simulink library "lib_controls"  (Simulink 7.9)
settings: Solver=ode45  SolverMode=SingleTasking  StartTime=0.0  StopTime=10.0  RelTol=1e-3
undefined symbols (not defined in the file or in its folder): amb_tmp, cs_charge_deplete_bool, cs_charge_pwr, cs_charge_trq, cs_clt_tmp, cs_decel_fc_off, cs_decel_regen_threshold, cs_dl_assist_trq_threshold, cs_dl_regen_trq_threshold, cs_electric_decel_spd, cs_electric_launch_spd, cs_electric_launch_spd_hi, cs_electric_launch_spd_lo, cs_eng_min_spd, cs_eng_on_soc, cs_fc_init_state, cs_fc_max_pwr_frac, cs_fc_min_pwr_frac, cs_fc_on, cs_fc_pwr_opt, cs_fc_spd_opt, cs_fuzzy_fuel_mode, cs_hi_soc, cs_hi_trq_frac, cs_lo_soc, cs_lo_trq_frac, cs_max_gc_spd, cs_max_pwr, cs_max_pwr_fall_rate, cs_max_pwr_rise_rate, cs_mc_assist_max_frac, cs_mc_assist_min_frac, cs_mc_assist_slope, cs_mc_regen_max_frac, cs_mc_regen_min_frac, cs_mc_regen_slope, cs_mean_eff, cs_mean_eff_bool, cs_min_gc_spd, cs_min_off_time, cs_min_pwr, cs_min_trq_frac, cs_mph_avg_time, cs_off_trq_frac, cs_plot_output, cs_pwr, cs_regen_avg_time, cs_scale_factor, cs_shutoff, cs_soc_range, cs_spd, cs_target_soc, cs_trq_to_soc_factor, cvt_locus_pwr, cvt_locus_spd, cyc_mph, enable_sim_stop_distance, enable_sim_stop_max_spd, enable_sim_stop_speed, enable_sim_stop_time ... (+110)
libraries: lib_controls x124, simulink3 x13, simulink x5, lib_etc x1
(part 8 of 17)

== system lib_controls/<vc> series/gearbox control for series  HV and EV ==
  note: default gear number
      | calculation
  note: default shifting
      | calculation
  note: default gear ratio
      | calculation
  note: local GOTO blocks:
  gb_trq_out_r : Inport
  gb_spd_out_r : Inport  Port=2
  prev. Pout/Pin : Inport  Port=3
  tires are at traction limit : Inport  Port=4
  Block NOTES : Subsystem
      mask Display: disp('Block\nNOTES')
  Constant : Constant
  Constant14 : Constant  Value=tx_speed_dep
  Constant15 : Constant  Value=tx_speed_dep
  Demux : Demux  Outputs=2
  Fcn : Fcn  Expr=1/u
  Fcn1 : Fcn  Expr=1/u
  Gain1 : Gain  Gain=-1  SaturateOnIntegerOverflow=on  OutDataTypeStr=Inherit: Same as input  ParamDataTypeStr=Inherit: Same as input
  MOTOR torque capability : Lookup  InputValues=mc_map_spd*mc_spd_scale  Table=mc_max_trq*mc_trq_scale+eps  SaturateOnIntegerOverflow=on
  Mux : Mux  Inputs=2
  Product2 : Product  Inputs=*/  SaturateOnIntegerOverflow=on  RndMeth=Zero  InputSameDT=on  OutDataTypeStr=Inherit: Same as first input
  Product3 : Product  SaturateOnIntegerOverflow=on  RndMeth=Zero  InputSameDT=on  OutDataTypeStr=Inherit: Same as first input
  Rate Limiter : RateLimiter  RisingSlewLimit=1/(gb_shift_delay+eps)  FallingSlewLimit=-1/(gb_shift_delay+eps)
  Saturation : Saturate  UpperLimit=1  LowerLimit=0.2
  Saturation1 : Saturate  UpperLimit=gb_gears_num  LowerLimit=1
  Speed Dependent Shifting : lib_controls/SubSystem/Speed Dependent Shifting
      settings: RTWFcnNameOpts=Auto  RTWFileNameOpts=Auto
  Switch : Switch  Threshold=eps  SaturateOnIntegerOverflow=on  InputSameDT=on
  Switch3 : Switch  Threshold=0.5  SaturateOnIntegerOverflow=on  InputSameDT=on
  Switch4 : Switch  Threshold=0.5  SaturateOnIntegerOverflow=on  InputSameDT=on
  allow downshift? : Subsystem
  current gear number : Sum  SaturateOnIntegerOverflow=on  InputSameDT=on  OutDataTypeStr=Inherit: Same as first input
  delta gear number : Switch  Threshold=eps  SaturateOnIntegerOverflow=on  InputSameDT=on
  downshift  command : Subsystem
  gb_spd_in_r : Product  SaturateOnIntegerOverflow=on  RndMeth=Zero  InputSameDT=on  OutDataTypeStr=Inherit: Same as first input
  gear ratio : Lookup  InputValues=[1:length(gb_ratio)]  Table=gb_ratio  SaturateOnIntegerOverflow=on
  gear ratio1 : Lookup  InputValues=[1:length(gb_ratio)]  Table=gb_ratio  SaturateOnIntegerOverflow=on
  gearbox speed estimator : Subsystem
  load=T/ (maxT at spd) : Saturate  UpperLimit=1  LowerLimit=0
  prev gear number : Memory  X0=1
  prev gear ratio : Memory  X0=gb_ratio(1)
  shifting1 : Subsystem
  upshift  command : Subsystem
  ~gb_trq_in_r : Product  Inputs=3  SaturateOnIntegerOverflow=on  RndMeth=Zero  InputSameDT=on  OutDataTypeStr=Inherit: Same as first input
  "gear number, out" : Outport  InitialOutput=0
  "gear ratio, out" : Outport  Port=2  InitialOutput=0
  "shifting, out" : Outport  Port=3  InitialOutput=0
  wires:
  gearbox speed estimator/1(Out1) -> MOTOR torque capability/1, downshift  command/3(engine speed), upshift  command/3(engine speed)
  gb_spd_in_r/1 -> gearbox speed estimator/1(gb_spd_in_r if no gear change)
  current gear number/1 -> Saturation1/1
  Saturation/1 -> Fcn/1
  prev. Pout/Pin/1 -> Saturation/1
  gb_trq_out_r/1 -> ~gb_trq_in_r/1
  upshift  command/1(command) -> delta gear number/1, delta gear number/2
  gear ratio/1 -> prev gear ratio/1
  Rate Limiter/1 -> gear ratio/1
  gb_spd_out_r/1 -> gb_spd_in_r/1
  downshift  command/1(command) -> Gain1/1
  Gain1/1 -> Product3/2
  Product3/1 -> delta gear number/3
  allow downshift?/1(allow shift) -> Product3/1
  prev gear ratio/1 -> Fcn1/1, gb_spd_in_r/2
  delta gear number/1 -> current gear number/2
  Fcn1/1 -> ~gb_trq_in_r/3
  MOTOR torque capability/1 -> Product2/2
  Product2/1 -> load=T/ (maxT at spd)/1
  ~gb_trq_in_r/1 -> Product2/1
  Fcn/1 -> ~gb_trq_in_r/2
  load=T/ (maxT at spd)/1 -> Switch/3
  tires are at traction limit/1 -> Switch/2
  Constant/1 -> Switch/1
  Switch/1 -> upshift  command/2(engine load), downshift  command/2(engine load)
  Saturation1/1 -> prev gear number/1, gear ratio1/1, shifting1/1(gear number), Rate Limiter/1, [def_gear_num]
  prev gear number/1 -> allow downshift?/1(prev gearnum), upshift  command/1(prev gear number), downshift  command/1(prev gear number), current gear number/1
  Constant14/1 -> Switch3/2
  [def_gear_num] -> Switch3/3
  Constant15/1 -> Switch4/2
  [spd_dep_muxed] -> Switch4/1
  Mux/1 -> Switch4/3
  [def_gear_ratio] -> Mux/1
  [def_shifting] -> Mux/2
  Switch4/1 -> Demux/1
  [spd_dep_gear_num] -> Switch3/1
  [v_req_limited] -> Speed Dependent Shifting/1
  Speed Dependent Shifting/1 -> [spd_dep_muxed]
  Speed Dependent Shifting/2 -> [spd_dep_gear_num]
  Demux/1 -> "gear ratio, out"/1
  Demux/2 -> "shifting, out"/1
  Switch3/1 -> "gear number, out"/1
  gear ratio1/1 -> [def_gear_ratio]
  shifting1/1(out_1) -> [def_shifting]

== system lib_controls/<vc> series/key_on ==
  Clock : Clock
  Fcn1 : Fcn  Expr=rem(u[1],period)
  Look-Up Table : Lookup  InputValues=t  Table=y  SaturateOnIntegerOverflow=on
  out_1 : Outport  InitialOutput=0
  wires:
  Look-Up Table/1 -> out_1/1
  Clock/1 -> Fcn1/1
  Fcn1/1 -> Look-Up Table/1

== system lib_controls/<vc> series/motor controller logic ==
  bus voltage : Inport
  req'd input power (W) : Inport  Port=2
  req'd output spd (rad/s) : Inport  Port=3
  shifting : Inport  Port=4
  Abs : Abs  SaturateOnIntegerOverflow=on
  Abs1 : Abs  SaturateOnIntegerOverflow=on
  Block NOTES : Subsystem
      mask Display: disp('Block\nNOTES')
  Constant : Constant  Value=mc_max_crrnt
  Constant1 : Constant  Value=0.001
  Constant2 : Constant  Value=0
  Logical Operator1 : Logic  Operator=NOT  Inputs=1
  Memory : Memory  X0=ess_module_num*mean(ess_voc(1,:))
  MinMax : MinMax  Inputs=2  SaturateOnIntegerOverflow=on  InputSameDT=on
  Product1 : Product  SaturateOnIntegerOverflow=on  RndMeth=Zero  InputSameDT=on  OutDataTypeStr=Inherit: Same as first input
  Relational Operator : RelationalOperator  Operator=<=  InputSameDT=on
  Relational Operator2 : RelationalOperator  Operator===  InputSameDT=on
  Sign : Subsystem
      mask Type: Sign
      mask Description: y = sign(x)
      mask Help: Sign Function:\n\t\t\ty = 1 if x > 0\n\t\t\ty = 0 if x = 0\n\t\t\ty = -1 if x < 0
      mask Display: plot(-50,-50,50,50,[-50,50],[0,0],[0,0],[-50,50],[-40,0],[-30,-30],[0,40],[30,30])
  Switch : Switch  Threshold=eps  SaturateOnIntegerOverflow=on  InputSameDT=on
  current-limited power : Product  SaturateOnIntegerOverflow=on  RndMeth=Zero  InputSameDT=on  OutDataTypeStr=Inherit: Same as first input
  true if motor should be shut down : Logic  Operator=OR
  req'd input power (W)1 : Outport  InitialOutput=0
  tag scope: mc_crrnt_limited=global
  wires:
  Abs1/1 -> Relational Operator/1
  true if motor should be shut down/1 -> Logical Operator1/1
  shifting/1 -> true if motor should be shut down/2
  Logical Operator1/1 -> Switch/2
  Constant/1 -> Product1/2
  Abs/1 -> MinMax/2
  Sign/1(out_1) -> current-limited power/2
  Constant2/1 -> Switch/3
  Switch/1 -> req'd input power (W)1/1
  current-limited power/1 -> Switch/1
  Product1/1 -> Relational Operator2/1, MinMax/1
  MinMax/1 -> current-limited power/1, Relational Operator2/2
  Relational Operator2/1 -> [mc_crrnt_limited]
  Relational Operator/1 -> true if motor should be shut down/1
  Constant1/1 -> Relational Operator/2
  req'd output spd (rad/s)/1 -> Abs1/1
  bus voltage/1 -> Memory/1
  Memory/1 -> Product1/1
  req'd input power (W)/1 -> Abs/1, Sign/1(in_1)

== system lib_controls/<vc> series/series 'clutch' control ==
  engine on : Inport
  Block NOTES : Subsystem
      mask Display: disp('Block\nNOTES')
  Clock : Clock
  Constant6 : Constant
  Constant7 : Constant  Value=3
  Memory1 : Memory  X0=cyc_mph(1,2)>0
  Memory2 : Memory  X0=-1
  Sum : Sum  Inputs=+-  SaturateOnIntegerOverflow=on  InputSameDT=on  OutDataTypeStr=Inherit: Same as first input
  Switch : Switch  Threshold=eps  SaturateOnIntegerOverflow=on  InputSameDT=on
  Switch1 : Switch  Threshold=0.5  SaturateOnIntegerOverflow=on  InputSameDT=on
  Transport Delay : TransportDelay  DelayTime=0.5
  clutch slipping1 : Logic
  clutch slipping2 : Logic
  clutch state : Outport
  wires:
  engine on/1 -> clutch slipping2/1, Transport Delay/1, Memory1/1, clutch slipping1/1
  Sum/1 -> Switch1/2
  Memory2/1 -> Sum/2
  Clock/1 -> Memory2/1, Sum/1
  clutch slipping2/1 -> Switch1/3
  Transport Delay/1 -> clutch slipping2/2
  clutch slipping1/1 -> Switch1/1
  Constant6/1 -> Switch/3
  Switch/1 -> clutch state/1
  Switch1/1 -> Switch/2
  Constant7/1 -> Switch/1
  Memory1/1 -> clutch slipping1/2

== system lib_controls/Adaptive control strategy <cs>/Delta SOC expected from regen ==
  "trq and spd req'd into clutch (N*m, rad/s)" : Inport
  "  1" : Constant  Value=0
  " 2" : Constant  Value=0
  Delta SOC : Sum  Inputs=-+  SaturateOnIntegerOverflow=on  InputSameDT=on  OutDataTypeStr=Inherit: Same as first input
  Logical Operator : Logic
  Memory1 : Memory  X0=ess_init_soc
  "Regen  (Tmc<0,  but Tfc<=0)" : Switch  Threshold=eps  SaturateOnIntegerOverflow=on  InputSameDT=on
  Regen flag conditions : Constant  Value=0
  Relational Operator : RelationalOperator  Operator=<=  InputSameDT=on
  Relational Operator1 : RelationalOperator  Operator=<  InputSameDT=on
  Saturation : Saturate  UpperLimit=1  LowerLimit=0
  Subsystem : Subsystem  mask(Running Average){n=cs_regen_avg_time}
      mask prompts: n "Averaging Time (s)"
      mask help: Running Average
      mask Help: Output is the average of the last (Averaging Time) seconds of input.
      mask Display: disp('Running\nAverage')
  trq : Selector  InputPortWidth=2  IndexOptions=Index vector (dialog)  Indices=1  OutputSizes=1
  Delta SOC regen : Outport
  wires:
  Delta SOC/1 -> Saturation/1
  "Regen  (Tmc<0,  but Tfc<=0)"/1 -> Subsystem/1(in_1)
  Subsystem/1(out_1) -> Delta SOC regen/1
  Logical Operator/1 -> "Regen  (Tmc<0,  but Tfc<=0)"/2
  [SOC] -> Delta SOC/2, Memory1/1
  Memory1/1 -> Delta SOC/1
  Saturation/1 -> "Regen  (Tmc<0,  but Tfc<=0)"/1
  "trq and spd req'd into clutch (N*m, rad/s)"/1 -> trq/1
  "  1"/1 -> "Regen  (Tmc<0,  but Tfc<=0)"/3
  trq/1 -> Relational Operator/1
  Relational Operator/1 -> Logical Operator/2
  Relational Operator1/1 -> Logical Operator/1
  Regen flag conditions/1 -> Relational Operator/2
  " 2"/1 -> Relational Operator1/2
  [mc_trq_out_a] -> Relational Operator1/1

== system lib_controls/Adaptive control strategy <cs>/Finds operation  point - energy/emissions  weighting ==
  "trq and spd req'd into clutch (N*m, rad/s)" : Inport
  Delta SOC expected from regen : Inport  Port=2
  Memory : Memory  X0=amb_tmp
  Memory1 : Memory  X0=amb_tmp
  Memory2 : Memory  X0=amb_tmp
  Minimize the  energy used  and emissions : Subsystem
  Mux2 : Mux  Inputs=7
  Subsystem : Subsystem  mask(Running Average){n=cs_mph_avg_time}
      mask prompts: n "Averaging Time (s)"
      mask help: Running Average
      mask Help: Output is the average of the last (Averaging Time) seconds of input.
      mask Display: disp('Running\nAverage')
  total fuel used (gal)1 : ToWorkspace  VariableName=cs_DeltaSOC_regen
      settings: MaxDataPoints=50000
  trq req'd from  engine (N*m) : Outport
  wires:
  Delta SOC expected from regen/1 -> total fuel used (gal)1/1, Mux2/2
  [ex_cat_tmp] -> Memory/1
  Memory/1 -> Mux2/6
  [cyc_mph_r] -> Subsystem/1(in_1)
  Subsystem/1(out_1) -> Mux2/4
  [SOC] -> Mux2/3
  [ess_tmp] -> Memory2/1
  Memory2/1 -> Mux2/7
  Mux2/1 -> Minimize the  energy used  and emissions/1(input vector)
  Minimize the  energy used  and emissions/1(Tfc) -> trq req'd from  engine (N*m)/1
  [fc_clt_tmp] -> Memory1/1
  Memory1/1 -> Mux2/5
  "trq and spd req'd into clutch (N*m, rad/s)"/1 -> Mux2/1

== system lib_controls/Fuzzy Logic control strategy <cs>/Block NOTES ==
  note: Where TLOAD is the load required from the drive cycle due to acceleration, drag, road grade, etc., and
      | TICE_Set is the desired output torque of the ICE.  The controller outputs the change of the throttle command.
  note: Due to the highly nonlinear, time varying nature of the plant, the control strategy will be
      |  implemented with the use of a fuzzy logic controller (FLC). The FLC will use two
      | inputs:  the battery pack SOC and the desired ICE torque. Based on the above inputs,
      | the ICE operating point is set (according to the MODE selected). Along the simulation,
      | in the reverse loop, the desired e-machine torque is calculated from the
      | following equation.
      |
      | TEM_Desired = TLOAD - TICE_Set
  note: The idea behind the Fuzzy Logic control strategy is to let the ICE run at an operating point
      | that consumes less than x gram of fuel per second at all operating conditions (FUSE USE MODE) or to
      | operate about a preak efficiency point (EFFICIENCY MODE).  Since an Electric Machine is available
      | to load-level, the HEV can use its e-machine to force the engine to operate in a region that consumes less fuel,
      | while maintaining  the state of charge (SOC) of the battery pack over the  majority of the drive cycle.
      | This is achieved by  using to E-Machine to compensate for the dearth in Torque required to meet the road load.
  note: This Block contains the Fuzzy Logic Control Strategy to control a parallel hybrid configuration.
      |
      | A standard set of inputs (SoC and ICE torque required) are input in the beginning. Then scaling is done
      | to the inputs to reflect the input membership functions. Likewise, the outputs are scaled based on the no. of output
      | membership functions. The above block diagram also calls the M-Function which contains the rules.

== system lib_controls/Fuzzy Logic control strategy <cs>/Fuzzy logic Code ==
  note: FUZZY LOGIC CODE
  Torque : Inport
  SoC : Inport  Port=2
  Block NOTES : Subsystem
      mask Display: disp('Block\nNOTES')
  Fuel use  or Efficieny : Switch  Threshold=eps  SaturateOnIntegerOverflow=on  InputSameDT=on
  MATLAB Fcn EFFICIENCY MODE : MATLABFcn  MATLABFcn=mfuzzy_eff_mode(u(1),u(2))  OutputDimensions=1
  MATLAB Fcn FUEL USE MODE : MATLABFcn  MATLABFcn=mfuzzy_fuel_mode(u(1),u(2))  OutputDimensions=1
  Mode switcher : Constant  Value=cs_fuzzy_fuel_mode
  Mux : Mux  Inputs=2
  delta  alpha : Outport
  wires:
  Mux/1 -> MATLAB Fcn FUEL USE MODE/1, MATLAB Fcn EFFICIENCY MODE/1
  Torque/1 -> Mux/1
  SoC/1 -> Mux/2
  Mode switcher/1 -> Fuel use  or Efficieny/2
  Fuel use  or Efficieny/1 -> delta  alpha/1
  MATLAB Fcn FUEL USE MODE/1 -> Fuel use  or Efficieny/1
  MATLAB Fcn EFFICIENCY MODE/1 -> Fuel use  or Efficieny/3

== system lib_controls/Fuzzy Logic control strategy <cs>/Input Scaling ==
  note: INPUT SCALING
  note: STANDARD INPUTS
  Torque required : Inport
  " 2" : Sum  SaturateOnIntegerOverflow=on  InputSameDT=on  OutDataTypeStr=Inherit: Same as first input
  " 3" : Sum  Inputs=+-  SaturateOnIntegerOverflow=on  InputSameDT=on  OutDataTypeStr=Inherit: Same as first input
  " 5" : Sum  SaturateOnIntegerOverflow=on  InputSameDT=on  OutDataTypeStr=Inherit: Same as first input
  " 6" : Sum  SaturateOnIntegerOverflow=on  InputSameDT=on  OutDataTypeStr=Inherit: Same as first input
  " 7" : Sum  Inputs=++-  SaturateOnIntegerOverflow=on  InputSameDT=on  OutDataTypeStr=Inherit: Same as first input
  Block NOTES : Subsystem
      mask Display: disp('Block\nNOTES')
  Constant5 : Constant  Value=5
  Constant6 : Constant
  Constant7 : Constant  Value=5
  Constant8 : Constant  Value=6
  Constant9 : Constant  Value=10e4*eps
  Product8 : Product  Inputs=**/  SaturateOnIntegerOverflow=on  RndMeth=Zero  InputSameDT=on  OutDataTypeStr=Inherit: Same as first input
  Relational Operator : RelationalOperator  Operator=<=  InputSameDT=on
  Saturation 1-11 : Saturate  UpperLimit=11  LowerLimit=1
  "Saturation 1-11 " : Saturate  UpperLimit=11  LowerLimit=1
  SoC scaling function 1-11 : Fcn  Expr=10*(u-cs_hi_soc)/(cs_hi_soc-cs_lo_soc)+11
  Switch1 : Switch  Threshold=eps  SaturateOnIntegerOverflow=on  InputSameDT=on
  Target ICE Line : Lookup  InputValues=fc_map_spd*fc_spd_scale  Table=flc_target*fc_trq_scale  SaturateOnIntegerOverflow=on
  epsilon : Constant  Value=eps
  max_torque lookup : Lookup  InputValues=fc_map_spd*fc_spd_scale  Table=fc_max_trq*fc_trq_scale  SaturateOnIntegerOverflow=on
  trouble : Product  Inputs=**/  SaturateOnIntegerOverflow=on  RndMeth=Zero  InputSameDT=on  OutDataTypeStr=Inherit: Same as first input
  Torque : Outport
  SoC : Outport  Port=2
  tag scope: FLC1=global
  wires:
  Relational Operator/1 -> Switch1/2
  Product8/1 -> " 2"/1
  Constant6/1 -> " 2"/2
  " 2"/1 -> Switch1/1
  " 3"/1 -> trouble/1
  Constant7/1 -> trouble/2
  Constant8/1 -> " 5"/2
  trouble/1 -> " 5"/1
  [SOC] -> SoC scaling function 1-11/1
  Saturation 1-11/1 -> SoC/1
  " 5"/1 -> Switch1/3
  "Saturation 1-11 "/1 -> Torque/1
  Constant5/1 -> Product8/2
  Constant9/1 -> " 7"/2
  epsilon/1 -> " 6"/1
  " 6"/1 -> Product8/3
  " 7"/1 -> trouble/3
  [engine_rpm] -> Target ICE Line/1, max_torque lookup/1
  SoC scaling function 1-11/1 -> Saturation 1-11/1
  Switch1/1 -> "Saturation 1-11 "/1
  max_torque lookup/1 -> " 7"/1
  Torque required/1 -> Product8/1, Relational Operator/1, " 3"/1
  Target ICE Line/1 -> [FLC1], Relational Operator/2, " 6"/2, " 3"/2, " 7"/3

== system lib_controls/Fuzzy Logic control strategy <cs>/Output scaling ==
  note: OUTPUT SCALING
  "delta alpha " : Inport
  " " : Sum  Inputs=+-  SaturateOnIntegerOverflow=on  InputSameDT=on  OutDataTypeStr=Inherit: Same as first input
  " 1" : Sum  Inputs=+-  SaturateOnIntegerOverflow=on  InputSameDT=on  OutDataTypeStr=Inherit: Same as first input
  " 2" : Sum  SaturateOnIntegerOverflow=on  InputSameDT=on  OutDataTypeStr=Inherit: Same as first input
  " 3" : Sum  Inputs=+-  SaturateOnIntegerOverflow=on  InputSameDT=on  OutDataTypeStr=Inherit: Same as first input
  Block NOTES : Subsystem
      mask Display: disp('Block\nNOTES')
  Constant : Constant  Value=6
  Constant1 : Constant
  Constant2 : Constant  Value=5
  Constant3 : Constant  Value=6
  Constant4 : Constant  Value=5
  Product4 : Product  SaturateOnIntegerOverflow=on  RndMeth=Zero  InputSameDT=on  OutDataTypeStr=Inherit: Same as first input
  Product5 : Product  Inputs=*/  SaturateOnIntegerOverflow=on  RndMeth=Zero  InputSameDT=on  OutDataTypeStr=Inherit: Same as first input
  Product6 : Product  SaturateOnIntegerOverflow=on  RndMeth=Zero  InputSameDT=on  OutDataTypeStr=Inherit: Same as first input
  Product7 : Product  Inputs=*/  SaturateOnIntegerOverflow=on  RndMeth=Zero  InputSameDT=on  OutDataTypeStr=Inherit: Same as first input
  Relational Operator : RelationalOperator  Operator=<=  InputSameDT=on
  Saturation 1-11 : Saturate  UpperLimit=11  LowerLimit=1
  Saturation4 : Saturate  UpperLimit=max(fc_max_trq*fc_trq_scale)  LowerLimit=0
  Switch1 : Switch  Threshold=eps  SaturateOnIntegerOverflow=on  InputSameDT=on
  max_torque lookup : Lookup  InputValues=fc_map_spd*fc_spd_scale  Table=fc_max_trq*fc_trq_scale  SaturateOnIntegerOverflow=on
  ICE Torque command : Outport
  wires:
  Constant/1 -> Relational Operator/2
  Constant1/1 -> " "/2
  Saturation 1-11/1 -> Relational Operator/1, " "/1
  " "/1 -> Product4/2
  Product4/1 -> Product5/1
  Constant2/1 -> Product5/2
  [FLC1] -> Product4/1, " 2"/2, " 3"/2
  "delta alpha "/1 -> " 1"/1, Saturation 1-11/1
  Constant3/1 -> " 1"/2
  " 1"/1 -> Product6/1
  " 3"/1 -> Product6/2
  Product6/1 -> Product7/1
  Constant4/1 -> Product7/2
  Product5/1 -> Switch1/1
  Relational Operator/1 -> Switch1/2
  " 2"/1 -> Switch1/3
  Product7/1 -> " 2"/1
  Switch1/1 -> Saturation4/1
  Saturation4/1 -> ICE Torque command/1
  [engine_rpm] -> max_torque lookup/1
  max_torque lookup/1 -> " 3"/1

== system lib_controls/Fuzzy Logic control strategy <cs>/help ==

== system lib_controls/Fuzzy Logic control strategy with Emissions <cs>/Block NOTES ==
  note: The Fuzzy Control Block takes in the torque and speed requested by the clutch (sink) and calculates
      | the torque split between the ICE and the Motor. The fuzzy logic algorithm sets a base (optimal)
      | operating point of the ICE and modifies the actual operating point about the optimal, based on
      | the actual torque request and the battery State of Charge (SOC). Finally, a torque request is sent to the
      | ICE and the motor buffers the remaining torque (positive or negative).

== system lib_controls/Fuzzy Logic control strategy with Emissions <cs>/Fuzzy logic Code ==
  note: FUZZY LOGIC CODE
  Torque : Inport
  SoC : Inport  Port=2
  Block NOTES : Subsystem
      mask Display: disp('Block\nNOTES')
  "MATLAB Fcn GPS " : MATLABFcn  MATLABFcn=mfuzzy_emissions(u(1),u(2))  OutputDimensions=1
  Mux : Mux  Inputs=2
  delta  alpha : Outport
  wires:
  Mux/1 -> "MATLAB Fcn GPS "/1
  Torque/1 -> Mux/1
  "MATLAB Fcn GPS "/1 -> delta  alpha/1
  SoC/1 -> Mux/2

== system lib_controls/Fuzzy Logic control strategy with Emissions <cs>/Input Scaling ==
  note: INPUTS
  note: INPUT SCALING
  note: Engine COLD
  note: Motor Max
      | Torque reached
  note: engine speed
  Torque required : Inport
  " 2" : Sum  SaturateOnIntegerOverflow=on  InputSameDT=on  OutDataTypeStr=Inherit: Same as first input
  " 3" : Sum  Inputs=+-  SaturateOnIntegerOverflow=on  InputSameDT=on  OutDataTypeStr=Inherit: Same as first input
  " 5" : Sum  SaturateOnIntegerOverflow=on  InputSameDT=on  OutDataTypeStr=Inherit: Same as first input
  " 6" : Sum  SaturateOnIntegerOverflow=on  InputSameDT=on  OutDataTypeStr=Inherit: Same as first input
  " 7" : Sum  Inputs=++-  SaturateOnIntegerOverflow=on  InputSameDT=on  OutDataTypeStr=Inherit: Same as first input
  Block NOTES : Subsystem
      mask Display: disp('Block\nNOTES')
  Constant5 : Constant  Value=5
  Constant6 : Constant
  Constant7 : Constant  Value=5
  Constant8 : Constant  Value=6
  Constant9 : Constant  Value=10e4*eps
  Gain : Gain  Gain=vc_fc_warm_tmp_frac  SaturateOnIntegerOverflow=on  OutDataTypeStr=Inherit: Same as input  ParamDataTypeStr=Inherit: Same as input
  MATLAB Fcn Target torque : MATLABFcn  MATLABFcn=fuzzy_target_compute_emissions(u(1),u(2),u(3))  OutputDimensions=1
  Memory : Memory
  Mux : Mux  Inputs=3
  Product8 : Product  Inputs=**/  SaturateOnIntegerOverflow=on  RndMeth=Zero  InputSameDT=on  OutDataTypeStr=Inherit: Same as first input
  Relational Operator : RelationalOperator  Operator=<=  InputSameDT=on
  Relational Operator5 : RelationalOperator  Operator=<  InputSameDT=on
  "Saturation 1-11 " : Saturate  UpperLimit=11  LowerLimit=1
  Switch1 : Switch  Threshold=eps  SaturateOnIntegerOverflow=on  InputSameDT=on
  To Workspace4 : ToWorkspace  VariableName=flc_opt_trq  SampleTime=-1
  To Workspace5 : ToWorkspace  VariableName=flc_max_trq  SampleTime=-1
  epsilon : Constant  Value=eps
  max_torque lookup : Lookup  InputValues=fc_map_spd*fc_spd_scale  Table=fc_max_trq*fc_trq_scale  SaturateOnIntegerOverflow=on
  product : Product  Inputs=**/  SaturateOnIntegerOverflow=on  RndMeth=Zero  InputSameDT=on  OutDataTypeStr=Inherit: Same as first input
  thermostat setting : Constant  Value=fc_tstat
  Torque : Outport
  tag scope: FLC1=global
  wires:
  Switch1/1 -> "Saturation 1-11 "/1
  " 7"/1 -> product/3
  " 6"/1 -> Product8/3
  epsilon/1 -> " 6"/1
  Constant9/1 -> " 7"/2
  Constant5/1 -> Product8/2
  "Saturation 1-11 "/1 -> Torque/1
  " 5"/1 -> Switch1/3
  product/1 -> " 5"/1
  Constant8/1 -> " 5"/2
  Constant7/1 -> product/2
  " 3"/1 -> product/1
  " 2"/1 -> Switch1/1
  Constant6/1 -> " 2"/2
  Product8/1 -> " 2"/1
  Relational Operator/1 -> Switch1/2
  MATLAB Fcn Target torque/1 -> To Workspace4/1, " 7"/3, " 3"/2, " 6"/2, Relational Operator/2, [FLC1]
  [engine_rpm] -> max_torque lookup/1, Mux/3
  Mux/1 -> MATLAB Fcn Target torque/1
  max_torque lookup/1 -> " 7"/1, To Workspace5/1
  Torque required/1 -> " 3"/1, Relational Operator/1, Product8/1
  [mc_trq_limited] -> Memory/1
  thermostat setting/1 -> Gain/1
  Gain/1 -> Relational Operator5/2
  [fc_clt_tmp] -> Relational Operator5/1
  Relational Operator5/1 -> Mux/1
  Memory/1 -> Mux/2

== system lib_controls/Fuzzy Logic control strategy with Emissions <cs>/Output scaling ==
  note: OUTPUT SCALING
  "delta alpha " : Inport
  " " : Sum  Inputs=+-  SaturateOnIntegerOverflow=on  InputSameDT=on  OutDataTypeStr=Inherit: Same as first input
  " 1" : Sum  Inputs=+-  SaturateOnIntegerOverflow=on  InputSameDT=on  OutDataTypeStr=Inherit: Same as first input
  " 2" : Sum  SaturateOnIntegerOverflow=on  InputSameDT=on  OutDataTypeStr=Inherit: Same as first input
  " 3" : Sum  Inputs=+-  SaturateOnIntegerOverflow=on  InputSameDT=on  OutDataTypeStr=Inherit: Same as first input
  Block NOTES : Subsystem
      mask Display: disp('Block\nNOTES')
  Constant : Constant  Value=6
  Constant1 : Constant
  Constant2 : Constant  Value=5
  Constant3 : Constant  Value=6
  Constant4 : Constant  Value=5
  Product4 : Product  SaturateOnIntegerOverflow=on  RndMeth=Zero  InputSameDT=on  OutDataTypeStr=Inherit: Same as first input
  Product5 : Product  Inputs=*/  SaturateOnIntegerOverflow=on  RndMeth=Zero  InputSameDT=on  OutDataTypeStr=Inherit: Same as first input
  Product6 : Product  SaturateOnIntegerOverflow=on  RndMeth=Zero  InputSameDT=on  OutDataTypeStr=Inherit: Same as first input
  Product7 : Product  Inputs=*/  SaturateOnIntegerOverflow=on  RndMeth=Zero  InputSameDT=on  OutDataTypeStr=Inherit: Same as first input
  Relational Operator : RelationalOperator  Operator=<=  InputSameDT=on
  Saturation 1-11 : Saturate  UpperLimit=11  LowerLimit=1
  Saturation4 : Saturate  UpperLimit=max(fc_max_trq*fc_trq_scale)  LowerLimit=0
  Switch1 : Switch  Threshold=eps  SaturateOnIntegerOverflow=on  InputSameDT=on
  max_torque lookup : Lookup  InputValues=fc_map_spd*fc_spd_scale  Table=fc_max_trq*fc_trq_scale  SaturateOnIntegerOverflow=on
  ICE Torque command : Outport
  wires:
  max_torque lookup/1 -> " 3"/1
  [engine_rpm] -> max_torque lookup/1
  Saturation4/1 -> ICE Torque command/1
  Switch1/1 -> Saturation4/1
  Product7/1 -> " 2"/1
  " 2"/1 -> Switch1/3
  Relational Operator/1 -> Switch1/2
  Product5/1 -> Switch1/1
  Constant4/1 -> Product7/2
  Product6/1 -> Product7/1
  " 3"/1 -> Product6/2
  " 1"/1 -> Product6/1
  Constant3/1 -> " 1"/2
  "delta alpha "/1 -> Saturation 1-11/1, " 1"/1
  [FLC1] -> " 3"/2, " 2"/2, Product4/1
  Constant2/1 -> Product5/2
  Product4/1 -> Product5/1
  " "/1 -> Product4/2
  Saturation 1-11/1 -> " "/1, Relational Operator/1
  Constant1/1 -> " "/2
  Constant/1 -> Relational Operator/2

== system lib_controls/Fuzzy Logic control strategy with Emissions <cs>/SoC  ==
  note: soc
  note: cs_hi_soc
  note: cs_lo_soc
  note: BASE SOC LIMITS
      | High= 0. 55
      | Low  = 0.45
  Block NOTES : Subsystem
      mask Display: disp('Block\nNOTES')
  Mux : Mux  Inputs=3
  Saturation 1-11 : Saturate  UpperLimit=11  LowerLimit=1
  SoC scaling function 1-11 : Fcn  Expr=10*(u(1)-u(2))/(u(2)-u(3))+11
  default = 0.45 : Constant  Value=cs_lo_soc
  default = 0.55 : Constant  Value=cs_hi_soc
  SoC : Outport
  wires:
  Mux/1 -> SoC scaling function 1-11/1
  [SOC] -> Mux/1
  default = 0.55/1 -> Mux/2
  default = 0.45/1 -> Mux/3
  SoC scaling function 1-11/1 -> Saturation 1-11/1
  Saturation 1-11/1 -> SoC/1

== system lib_controls/Insight electric assist control strategy <cs> DIRECT SPLIT/1st gear ? ==
  note: 1st Gear
  In 1 : Inport
  In 2 : Inport  Port=2
  Constant : Constant  Value=125
  Constant1 : Constant
  Logical Operator : Logic
  Relational Operator1 : RelationalOperator  Operator===  InputSameDT=on
  Relational Operator2 : RelationalOperator  Operator=<  InputSameDT=on
  Switch11 : Switch  Threshold=eps  SaturateOnIntegerOverflow=on  InputSameDT=on
  Out1 : Outport
  wires:
  In 2/1 -> Switch11/1
  In 1/1 -> Switch11/3
  Constant1/1 -> Relational Operator1/2
  [gear_number] -> Relational Operator1/1
  Switch11/1 -> Out1/1
  Constant/1 -> Relational Operator2/2
  [cs_trq_in_r] -> Relational Operator2/1
  Relational Operator2/1 -> Logical Operator/2
  Logical Operator/1 -> Switch11/2
  Relational Operator1/1 -> Logical Operator/1

== system lib_controls/Insight electric assist control strategy <cs> DIRECT SPLIT/Alternator Function ==
  note: current speed (rad/s)
  note: Torque request
  In1 : Inport
  In2 : Inport  Port=2
  Block NOTES : Subsystem
      mask Display: disp('Block\nNOTES')
  Constant1 : Constant  Value=0
  Constant2 : Constant  Value=0
  Constant3 : Constant  Value=0
  Product : Product  Inputs=*/  SaturateOnIntegerOverflow=on  RndMeth=Zero  InputSameDT=on  OutDataTypeStr=Inherit: Same as first input
  Product1 : Product  Inputs=*/  SaturateOnIntegerOverflow=on  RndMeth=Zero  InputSameDT=on  OutDataTypeStr=Inherit: Same as first input
  Relational Operator1 : RelationalOperator  Operator===  InputSameDT=on
  Relational Operator6 : RelationalOperator  Operator=>  InputSameDT=on
  Sum{2..5} (4 alike) : Sum  Inputs=+-  SaturateOnIntegerOverflow=on  InputSameDT=on  OutDataTypeStr=Inherit: Same as first input
  Sum7 : Sum  Inputs=--  SaturateOnIntegerOverflow=on  InputSameDT=on  OutDataTypeStr=Inherit: Same as first input
  Switch1 : Switch  Threshold=eps  SaturateOnIntegerOverflow=on  InputSameDT=on
  Switch8 : Switch  Threshold=eps  SaturateOnIntegerOverflow=on  InputSameDT=on
  motor/controller input power map (W) only base torque : Lookup2D  RowIndex=mc_map_spd*mc_spd_scale  ColumnIndex=mc_map_trq*mc_trq_scale  Table=mc_inpwr_map*mc_spd_scale*mc_trq_scale  SaturateOnIntegerOverflow=on  InputSameDT=on
  motor/controller input power map (W) with REGEN : Lookup2D  RowIndex=mc_map_spd*mc_spd_scale  ColumnIndex=mc_map_trq*mc_trq_scale  Table=mc_inpwr_map*mc_spd_scale*mc_trq_scale  SaturateOnIntegerOverflow=on  InputSameDT=on
  prevent  divide by zero error : Saturate  UpperLimit=max(fc_spd_scale*fc_map_spd)  LowerLimit=vc_idle_spd
  prevent  divide by zero error2 : Saturate  UpperLimit=max(fc_spd_scale*fc_map_spd)  LowerLimit=vc_idle_spd
  saturation : Saturate  UpperLimit=inf  LowerLimit=0
  Motor torque : Outport
  alternator torque : Outport  Port=2
  wires:
  [acc_elec_pwr_est] -> Product/1
  Relational Operator6/1 -> Switch8/2
  Constant3/1 -> Relational Operator6/2
  prevent  divide by zero error2/1 -> Product1/2, motor/controller input power map (W) only base torque/1, motor/controller input power map (W) with REGEN/1
  [acc_elec_pwr_est] -> Sum5/1
  In2/1 -> prevent  divide by zero error2/1
  Sum2/1 -> motor/controller input power map (W) with REGEN/2, Sum3/1
  In1/1 -> motor/controller input power map (W) only base torque/2, Sum2/1, Switch8/1, Relational Operator6/1, Relational Operator1/1
  Sum5/1 -> saturation/1
  saturation/1 -> Product1/1
  motor/controller input power map (W) with REGEN/1 -> Sum4/2
  Sum4/1 -> Sum5/2
  prevent  divide by zero error/1 -> Product/2
  [engine_rpm] -> prevent  divide by zero error/1
  Switch8/1 -> Motor torque/1
  Product/1 -> Sum2/2, Sum7/2
  Sum7/1 -> alternator torque/1
  Sum3/1 -> Switch8/3
  Product1/1 -> Sum3/2, Sum7/1
  Constant1/1 -> Relational Operator1/2
  Relational Operator1/1 -> Switch1/2
  motor/controller input power map (W) only base torque/1 -> Switch1/3
  Constant2/1 -> Switch1/1
  Switch1/1 -> Sum4/1

== system lib_controls/Insight electric assist control strategy <cs> DIRECT SPLIT/Block NOTES ==
  note: HONDA INSIGHT TORQUE SPLIT CONTROL STRATEGY
      |
      | The Honda Insight Control Startegy is modeled in this block. The Input is the Torque and speed
      | required into the clutch. The electric motor torque contibution is then calculated based on the
      | following parameters:
      | 1. Acceleration torque
      | 2. Deceleration torque
      | 3. 1st gear selection
      | 4. Vehicle speed
      | etc...
      |
      | The electric motor is also the alternator in the vehicle. Thus, it produces the power required by the
      | accessory loads. The remaining is then demanded from the IC Engine. The 2 signals are then
      | sent to the respective blocks in the INSIGHT Model.

== system lib_controls/Insight electric assist control strategy <cs> DIRECT SPLIT/Clutch Engaged ? ==
  note: clutch not
      | disengaged
  note: Any torque
      |  requested from
      | Electric Motor
      | only when
      | clutch engaged
  In1 : Inport
  In2 : Inport  Port=2
  Constant2 : Constant
  Constant3 : Constant
  Constant4 : Constant  Value=0
  Logical Operator : Logic  Operator=NOT
  Relational Operator2 : RelationalOperator  Operator===  InputSameDT=on
  Relational Operator3 : RelationalOperator  Operator===  InputSameDT=on
  Switch2 : Switch  Threshold=eps  SaturateOnIntegerOverflow=on  InputSameDT=on
  Switch3 : Switch  Threshold=eps  SaturateOnIntegerOverflow=on  InputSameDT=on
  Out1 : Outport
  wires:
  Relational Operator2/1 -> Logical Operator/1
  [clutch_state] -> Relational Operator2/1
  Constant2/1 -> Relational Operator2/2
  Constant3/1 -> Relational Operator3/2
  Relational Operator3/1 -> Switch3/2
  Constant4/1 -> Switch3/3
  Switch3/1 -> Switch2/3
  In2/1 -> Switch3/1
  [engine_on] -> Relational Operator3/1
  Logical Operator/1 -> Switch2/2
  In1/1 -> Switch2/1
  Switch2/1 -> Out1/1

== system lib_controls/Insight electric assist control strategy <cs> DIRECT SPLIT/Hard Acceleration ==
  note: Transient = 1
  note: moderate
      | accn
  note: Insight max. effort Torque from motor
      | will be the minimum between
      | {6000 W/shaft_speed} Nm AND
      | the maximum output torque of motor (Nm)
  In1 : Inport
  In2 : Inport  Port=2
  Constant : Constant  Value=125
  Constant1 : Constant  Value=6000*mc_trq_scale
  Constant2 : Constant  Value=max(mc_max_trq)*mc_trq_scale
  Constant6 : Constant  Value=cs_dl_assist_trq_threshold
  Constant7 : Constant  Value=.3
  Define the Assist Characteristics : Fcn  Expr=cs_mc_assist_slope*(u-cs_dl_assist_trq_threshold)+ (cs_mc_assist_min_frac*max(mc_max_trq*mc_trq_scale))
  Derivative : Derivative
  Logical Operator : Logic
  MinMax : MinMax  Inputs=2  SaturateOnIntegerOverflow=on  InputSameDT=on
  Product1 : Product  Inputs=*/  SaturateOnIntegerOverflow=on  RndMeth=Zero  InputSameDT=on  OutDataTypeStr=Inherit: Same as first input
  Relational Operator2 : RelationalOperator  Operator=>  InputSameDT=on
  Relational Operator5 : RelationalOperator  InputSameDT=on
  Relational Operator6 : RelationalOperator  InputSameDT=on
  Saturate motor torque at approx 32% max trq : Saturate  UpperLimit=max(mc_max_trq*mc_trq_scale)*cs_mc_assist_max_frac  LowerLimit=min(mc_max_gen_trq*mc_trq_scale)
  Switch10 : Switch  Threshold=eps  SaturateOnIntegerOverflow=on  InputSameDT=on
  Switch2 : Switch  Threshold=eps  SaturateOnIntegerOverflow=on  InputSameDT=on
  "filter from divide by zero  or negative " : lib_etc/filter from divide by zero  or negative 
      settings: RTWFcnNameOpts=Auto  RTWFileNameOpts=Auto
  Out1 : Outport
  wires:
  Constant7/1 -> Relational Operator6/2
  Derivative/1 -> Relational Operator6/1
  Switch10/1 -> Switch2/3
  In2/1 -> Switch10/3
  Logical Operator/1 -> Switch10/2
  Relational Operator5/1 -> Logical Operator/1
  Relational Operator6/1 -> Logical Operator/2
  Define the Assist Characteristics/1 -> Saturate motor torque at approx 32% max trq/1
  Saturate motor torque at approx 32% max trq/1 -> Switch10/1
  Constant6/1 -> Relational Operator5/2
  In1/1 -> Relational Operator5/1, Define the Assist Characteristics/1, Relational Operator2/1
  [v_req_limited] -> Derivative/1
  Constant/1 -> Relational Operator2/2
  Constant1/1 -> Product1/1
  Relational Operator2/1 -> Switch2/2
  Switch2/1 -> Out1/1
  "filter from divide by zero  or negative "/1 -> Product1/2
  [fc_spd_est] -> "filter from divide by zero  or negative "/1
  MinMax/1 -> Switch2/1
  Product1/1 -> MinMax/2
  Constant2/1 -> MinMax/1

== system lib_controls/Insight electric assist control strategy <cs> DIRECT SPLIT/Hard Deceleration ==
  note: heavy decel
  note: light decel
  In1 : Inport
  Constant3 : Constant  Value=cs_dl_regen_trq_threshold
  Constant4 : Constant  Value=cs_dl_regen_trq_threshold
  Constant5 : Constant  Value=0
  Constant7 : Constant  Value=0
  Define regenerative  capabilities : Fcn  Expr=(u-cs_dl_regen_trq_threshold)*cs_mc_regen_slope + (cs_mc_regen_min_frac*min(mc_max_gen_trq*mc_trq_scale))
  Logical Operator : Logic
  Relational Operator3 : RelationalOperator  Operator=<=  InputSameDT=on
  Relational Operator4 : RelationalOperator  Operator=<  InputSameDT=on
  Relational Operator5 : RelationalOperator  Operator=>  InputSameDT=on
  Saturate motor torque at 100% max regen trq : Saturate  UpperLimit=max(mc_max_trq*mc_trq_scale)  LowerLimit=min(mc_max_gen_trq*mc_trq_scale)*cs_mc_regen_max_frac
  Switch10 : Switch  Threshold=eps  SaturateOnIntegerOverflow=on  InputSameDT=on
  Switch9 : Switch  Threshold=eps  SaturateOnIntegerOverflow=on  InputSameDT=on
  Out1 : Outport
  wires:
  Saturate motor torque at 100% max regen trq/1 -> Switch9/1
  Define regenerative  capabilities/1 -> Saturate motor torque at 100% max regen trq/1
  In1/1 -> Define regenerative  capabilities/1, Relational Operator3/1, Relational Operator4/1, Relational Operator5/1, Switch10/1
  Relational Operator3/1 -> Switch9/2
  Constant3/1 -> Relational Operator3/2
  Constant5/1 -> Relational Operator4/2
  Constant4/1 -> Relational Operator5/2
  Relational Operator4/1 -> Logical Operator/1
  Relational Operator5/1 -> Logical Operator/2
  Switch9/1 -> Out1/1
  Constant7/1 -> Switch10/3
  Logical Operator/1 -> Switch10/2
  Switch10/1 -> Switch9/3

== system lib_controls/Insight electric assist control strategy <cs> DIRECT SPLIT/No EM activity at Slow Speed ==
  note: slow
      | speed
  In1 : Inport
  Constant : Constant  Value=125
  Constant11 : Constant  Value=0
  Constant9 : Constant  Value=cs_decel_regen_threshold
  Logical Operator : Logic
  Relational Operator1 : RelationalOperator  Operator=<  InputSameDT=on
  Relational Operator7 : RelationalOperator  Operator=<  InputSameDT=on
  Switch4 : Switch  Threshold=eps  SaturateOnIntegerOverflow=on  InputSameDT=on
  m/s-->mph : Gain  Gain=1/0.447  SaturateOnIntegerOverflow=on  OutDataTypeStr=Inherit: Same as input  ParamDataTypeStr=Inherit: Same as input
  Out1 : Outport
  wires:
  Constant9/1 -> Relational Operator7/2
  [v_req_limited] -> m/s-->mph/1
  m/s-->mph/1 -> Relational Operator7/1
  In1/1 -> Switch4/3
  Switch4/1 -> Out1/1
  Constant11/1 -> Switch4/1
  Constant/1 -> Relational Operator1/2
  [cs_trq_in_r] -> Relational Operator1/1
  Logical Operator/1 -> Switch4/2
  Relational Operator7/1 -> Logical Operator/1
  Relational Operator1/1 -> Logical Operator/2

== system lib_controls/Insight electric assist control strategy <cs> DIRECT SPLIT/SoC Correction ==
  note: ORIGINAL TORQUE SIGNAL
  In1 : Inport
  16% of peak torque : Saturate  UpperLimit=0.16*15  LowerLimit=min(mc_max_gen_trq*mc_trq_scale)
  Block NOTES : Subsystem
      mask Display: disp('Block\nNOTES')
  Constant10 : Constant  Value=0.235
  Constant5 : Constant  Value=0.8
  Constant6 : Constant  Value=0.2
  Constant7 : Constant  Value=0.235
  Constant8 : Constant  Value=0.2
  Constant9 : Constant  Value=0.355
  Limited assist : MinMax  Inputs=2  SaturateOnIntegerOverflow=on  InputSameDT=on
  Low SoC : Logic
  Moderately low SoC : Logic
  No Assist : Saturate  UpperLimit=0  LowerLimit=min(mc_max_gen_trq*mc_trq_scale)
  Relational Operator6 : RelationalOperator  Operator=<=  InputSameDT=on
  Relational Operator7 : RelationalOperator  Operator=>  InputSameDT=on
  Relational Operator8 : RelationalOperator  Operator=<=  InputSameDT=on
  Relational Operator9 : RelationalOperator  Operator=>  InputSameDT=on
  Switch{4..7} (4 alike) : Switch  Threshold=eps  SaturateOnIntegerOverflow=on  InputSameDT=on
  Torque limiter : Fcn  Expr=u*6.88-1.4528
  Very high SoC : RelationalOperator  InputSameDT=on
  Very low SoC : RelationalOperator  Operator=<=  InputSameDT=on
  estimated peak torque : Gain  Gain=15  SaturateOnIntegerOverflow=on  OutDataTypeStr=Inherit: Same as input  ParamDataTypeStr=Inherit: Same as input
  no regen only assist : Saturate  UpperLimit=max(mc_max_trq*mc_trq_scale)  LowerLimit=0
  saturation : Saturate  UpperLimit=max(mc_max_trq*mc_trq_scale)  LowerLimit=min(mc_max_gen_trq*mc_trq_scale)
  Out1 : Outport
  wires:
  In1/1 -> Switch5/3, No Assist/1, 16% of peak torque/1, Limited assist/2, no regen only assist/1
  16% of peak torque/1 -> Switch6/1
  Torque limiter/1 -> estimated peak torque/1
  [SOC] -> Torque limiter/1, Very low SoC/1, Relational Operator7/1, Relational Operator6/1, Relational Operator9/1, Relational Operator8/1, Very high SoC/1
  No Assist/1 -> Switch5/1
  Very low SoC/1 -> Switch5/2
  Constant6/1 -> Very low SoC/2
  Constant8/1 -> Relational Operator7/2
  Constant7/1 -> Relational Operator6/2
  Relational Operator7/1 -> Moderately low SoC/2
  Relational Operator6/1 -> Moderately low SoC/1
  Switch5/1 -> Switch6/3
  Moderately low SoC/1 -> Switch6/2
  Switch6/1 -> Switch7/3
  Low SoC/1 -> Switch7/2
  Constant10/1 -> Relational Operator9/2
  Constant9/1 -> Relational Operator8/2
  no regen only assist/1 -> Switch4/1
  Very high SoC/1 -> Switch4/2
  Constant5/1 -> Very high SoC/2
  estimated peak torque/1 -> Limited assist/1
  Relational Operator9/1 -> Low SoC/2
  Relational Operator8/1 -> Low SoC/1
  Switch4/1 -> Out1/1
  Limited assist/1 -> Switch7/1
  Switch7/1 -> saturation/1
  saturation/1 -> Switch4/3

== system lib_controls/Insight electric assist control strategy <cs> DIRECT SPLIT/help ==

== system lib_controls/SubSystem/Speed Dependent Shifting ==
  note: SPEED
      | DEPENDENT
      | SHIFT
      | SIGNAL
  note: delta speed
  note: decel
      | case
  note: accel
      | case
  note: accel case
  note: decel case
  note: storing shifting and gear ratio
      | information to workspace
  "velocity required (limited) " : Inport
  Look-Up Table (gear for downshift) : Lookup  InputValues="tx_spd_dep_dnshift(:,1)   % vector of speeds m/s"  Table="tx_spd_dep_dnshift(:,2)  % gear number--must be step function"  SaturateOnIntegerOverflow=on
  Look-Up Table (gear for upshift) : Lookup  InputValues="tx_spd_dep_upshift(:,1)   % vector of speeds in m/s"  Table="tx_spd_dep_upshift(:,2)  % gear number--must be step function"  SaturateOnIntegerOverflow=on
  Mux : Mux  Inputs=2
  Mux2 : Mux  Inputs=2
  New gear ratio : ToWorkspace  VariableName=new_gear_ratio
      settings: MaxDataPoints=50000
  Rounding Function : Rounding  Operator=round
  Rounding Function1 : Rounding  Operator=round
  Saturation4 : Saturate  UpperLimit=gb_gears_num  LowerLimit=1
  Saturation5 : Saturate  UpperLimit=gb_gears_num  LowerLimit=1
  "delta speed (\"+\" is acceleration)" : Sum  Inputs=-+  SaturateOnIntegerOverflow=on  InputSameDT=on  OutDataTypeStr=Inherit: Same as first input
  gear ratio6 : Lookup  InputValues=[1:length(gb_ratio)]  Table=gb_ratio  SaturateOnIntegerOverflow=on
  gear ratio8 : Lookup  InputValues=[1:length(gb_ratio)]  Table=gb_ratio  SaturateOnIntegerOverflow=on
  prev veh speed : Memory  X0=1
  shifting : lib_controls/SubSystem/shifting
      settings: RTWFcnNameOpts=Auto  RTWFileNameOpts=Auto
  shifting1 : lib_controls/SubSystem/shifting
      settings: RTWFcnNameOpts=Auto  RTWFileNameOpts=Auto
  switch for gear number : Switch  Threshold=eps  SaturateOnIntegerOverflow=on  InputSameDT=on
  switch for gear ratio and shifting (muxed) : Switch  Threshold=eps  SaturateOnIntegerOverflow=on  InputSameDT=on
  total fuel used (gal) : ToWorkspace  VariableName=neg_gear_num
      settings: MaxDataPoints=50000
  gear ratio and shifting : Outport
  gear number : Outport  Port=2
  wires:
  "velocity required (limited) "/1 -> prev veh speed/1, "delta speed (\"+\" is acceleration)"/2, Look-Up Table (gear for downshift)/1, Look-Up Table (gear for upshift)/1
  prev veh speed/1 -> "delta speed (\"+\" is acceleration)"/1
  Mux2/1 -> switch for gear ratio and shifting (muxed)/3
  Mux/1 -> switch for gear ratio and shifting (muxed)/1
  shifting/1 -> Mux2/2
  gear ratio8/1 -> Mux2/1
  Saturation5/1 -> switch for gear number/3, total fuel used (gal)/1, gear ratio8/1, shifting/1
  gear ratio6/1 -> Mux/1
  shifting1/1 -> Mux/2
  Saturation4/1 -> switch for gear number/1, shifting1/1, gear ratio6/1
  switch for gear ratio and shifting (muxed)/1 -> New gear ratio/1, gear ratio and shifting/1
  switch for gear number/1 -> gear number/1
  "delta speed (\"+\" is acceleration)"/1 -> switch for gear number/2, switch for gear ratio and shifting (muxed)/2
  Look-Up Table (gear for upshift)/1 -> Rounding Function/1
  Rounding Function/1 -> Saturation4/1
  Look-Up Table (gear for downshift)/1 -> Rounding Function1/1
  Rounding Function1/1 -> Saturation5/1

== system lib_controls/SubSystem/braking strategy ==
  req'd speed (m/s) : Inport
  slip-limited force req'd (N) : Inport  Port=2
  Block NOTES : Subsystem
      mask Display: disp('Block\nNOTES')
  Constant : Constant  Value=0
  Constant1 : Constant
  Constant2 : Constant  Value=0
  Keep frac>0 : Saturate  UpperLimit=1  LowerLimit=0
  Product : Product  SaturateOnIntegerOverflow=on  RndMeth=Zero  InputSameDT=on  OutDataTypeStr=Inherit: Same as first input
  Product1 : Product  SaturateOnIntegerOverflow=on  RndMeth=Zero  InputSameDT=on  OutDataTypeStr=Inherit: Same as first input
  Sum : Sum  Inputs=--+  SaturateOnIntegerOverflow=on  InputSameDT=on  OutDataTypeStr=Inherit: Same as first input
  Switch : Switch  SaturateOnIntegerOverflow=on  InputSameDT=on
  Switch1 : Switch  SaturateOnIntegerOverflow=on  InputSameDT=on
  convert (mph) : Gain  Gain=2.2371  SaturateOnIntegerOverflow=on  OutDataTypeStr=Inherit: Same as input  ParamDataTypeStr=Inherit: Same as input
  front driveline braking fraction : Lookup  InputValues=wh_fa_dl_brake_mph  Table=wh_fa_dl_brake_frac  SaturateOnIntegerOverflow=on
  front friction braking fraction : Lookup  InputValues=wh_fa_fric_brake_mph  Table=wh_fa_fric_brake_frac  SaturateOnIntegerOverflow=on
  req'd front brake force (N) : Outport  InitialOutput=0
  req'd rear brake force (N) : Outport  Port=2  InitialOutput=0
  wires:
  Keep frac>0/1 -> Product1/2
  Sum/1 -> Keep frac>0/1
  Constant/1 -> Switch/1
  Product/1 -> Switch/3
  slip-limited force req'd (N)/1 -> Switch/2, Product/1, Product1/1, Switch1/2
  Switch/1 -> req'd front brake force (N)/1
  Product1/1 -> Switch1/3
  Constant2/1 -> Switch1/1
  Switch1/1 -> req'd rear brake force (N)/1
  req'd speed (m/s)/1 -> convert (mph)/1
  convert (mph)/1 -> front friction braking fraction/1, front driveline braking fraction/1
  front driveline braking fraction/1 -> Sum/2
  front friction braking fraction/1 -> Product/2, Sum/1
  Constant1/1 -> Sum/3

== system lib_controls/SubSystem/config traction control ==
  time-average vehicle speed  req'd (m/s) : Inport
  vehicle speed at beginning of time  step (m/s) : Inport  Port=2
  total tractive force req'd (N) : Inport  Port=3
  traction control 2 axle : lib_controls/SubSystem/traction control 2 axle
      settings: RTWFcnNameOpts=Auto  RTWFileNameOpts=Auto
  req'd force (N) : Outport
  req'd speed (m/s) : Outport  Port=2
  weight on front axle (N) : Outport  Port=3
  weight on rear axle (N) : Outport  Port=4
  front/total  traction ratio : Outport  Port=5
  wires:
  time-average vehicle speed  req'd (m/s)/1 -> traction control 2 axle/1
  vehicle speed at beginning of time  step (m/s)/1 -> traction control 2 axle/2
  total tractive force req'd (N)/1 -> traction control 2 axle/3
  traction control 2 axle/1 -> req'd force (N)/1
  traction control 2 axle/2 -> req'd speed (m/s)/1
  traction control 2 axle/3 -> weight on front axle (N)/1
  traction control 2 axle/4 -> weight on rear axle (N)/1
  traction control 2 axle/5 -> front/total  traction ratio/1

== system lib_controls/SubSystem/current veh mass (kg) ==
  Constant12 : Constant  Value=veh_mass
  Sum8 : Sum  Inputs=|++  SaturateOnIntegerOverflow=on  InputSameDT=on  OutDataTypeStr=Inherit: Same as first input
  Out1 : Outport
  wires:
  Sum8/1 -> Out1/1
  [veh_cargo_mass] -> Sum8/1
  Constant12/1 -> Sum8/2
